simulink model "mathmodelsim"  (R2024b)
settings: Solver=VariableStepAuto  StartTime=0.0  StopTime=10  RelTol=1e-3
undefined symbols (not defined in the file): angles, initial_height, jointstiffnes_damping, limits, plane_x, plane_y, plane_z, torque, X, Y, Z
libraries: sm_lib x162, nesl_utility x70, simulink x9, rllib x1
(part 1 of 5)
settings Model: Creator=User  LastModifiedBy=User

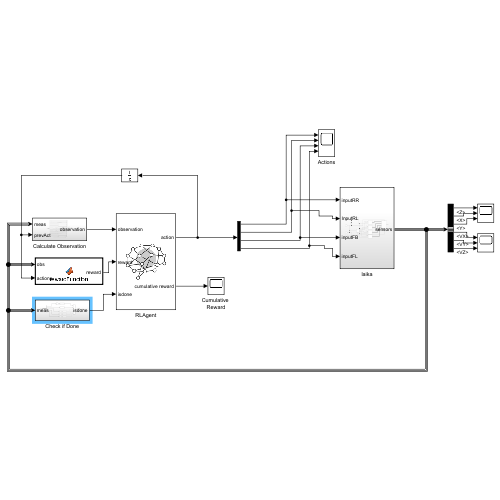
[thumbnail: Simulink's stored preview of the top-level diagram]
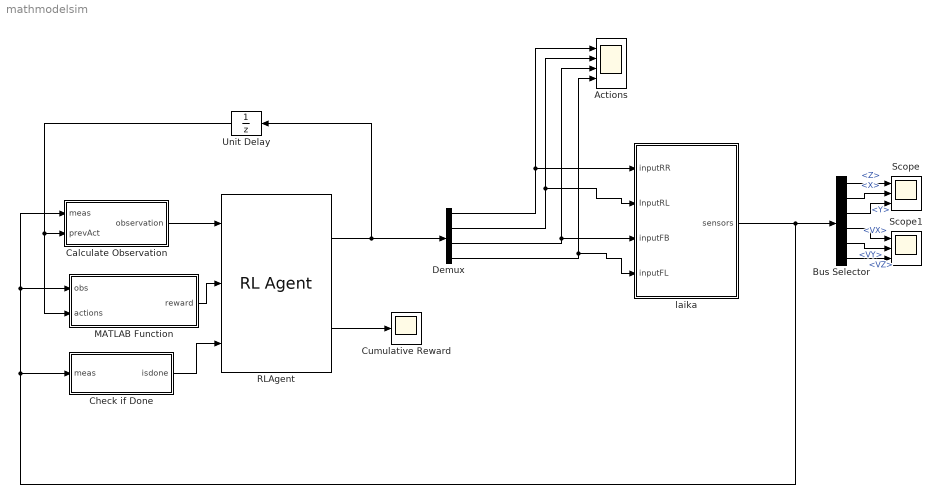
== system mathmodelsim ==
  Actions : Scope  NumInputPorts=4
  Bus Selector : BusSelector  OutputSignals=Z,X,Y,VX,VY,VZ
  Calculate Observation : Subsystem
  Check if Done : Subsystem
  Cumulative Reward : Scope
  Demux : Demux
  MATLAB Function : MATLAB Function  TreatAsAtomicUnit=on
  RLAgent : rllib/RL Agent  Agent=agent  ExternalActionAsInput=off  ProvideLastAction=off  ProvideCumRwd=on  TreatAsDirectFeedthrough=on  UseStrictObservationDataTypes=off
  Scope : Scope  NumInputPorts=3
  Scope1 : Scope  NumInputPorts=3
  Unit Delay : UnitDelay  SampleTime=-1  HasFrameUpgradeWarning=on
  laika : Subsystem
  wires:
  Bus Selector/1 -> Scope/1  "<Z>"
  Bus Selector/2 -> Scope/2  "<X>"
  Bus Selector/3 -> Scope/3  "<Y>"
  Bus Selector/4 -> Scope1/1  "<VX>"
  Bus Selector/5 -> Scope1/2  "<VY>"
  Bus Selector/6 -> Scope1/3  "<VZ>"
  Demux/3 -> Actions/3, laika/3(inputFB)
  RLAgent/2 -> Cumulative Reward/1
  Demux/2 -> laika/2(InputRL), Actions/2
  Demux/1 -> laika/1(inputRR), Actions/1
  Unit Delay/1 -> MATLAB Function/2(actions), Calculate Observation/2(prevAct)
  Demux/4 -> laika/4(inputFL), Actions/4
  MATLAB Function/1(reward) -> RLAgent/2
  Check if Done/1(isdone) -> RLAgent/3
  Calculate Observation/1(observation) -> RLAgent/1
  laika/1(sensors) -> Calculate Observation/1(meas), MATLAB Function/1(obs), Check if Done/1(meas), Bus Selector/1
  RLAgent/1 -> Demux/1, Unit Delay/1

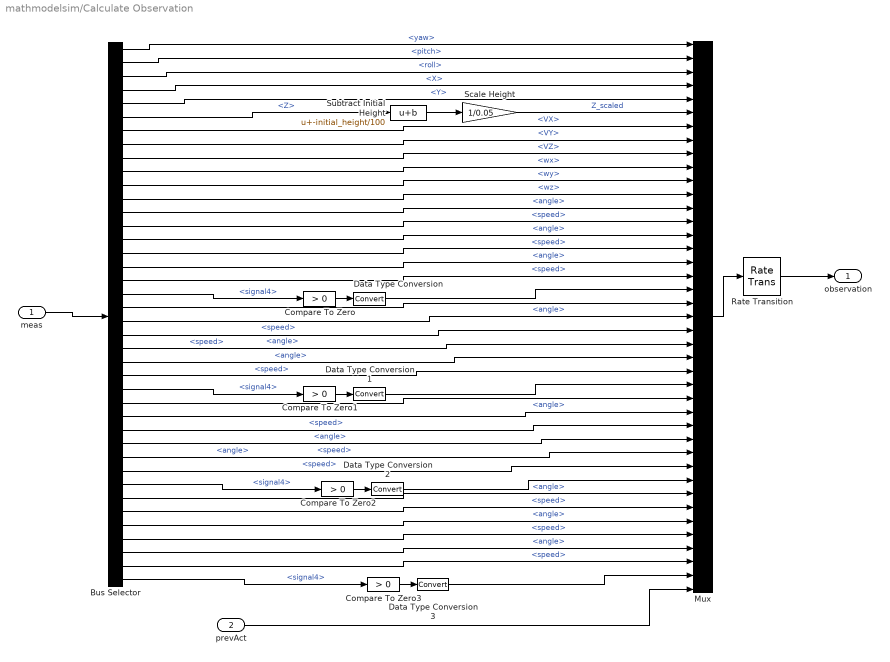
== system mathmodelsim/Calculate Observation ==
  meas : Inport
  prevAct : Inport  Port=2
  Bus Selector : BusSelector  OutputSignals=yaw,pitch,roll,X,Y,Z,VX,VY,VZ,wx,wy,wz,measRF.signal1.angle,measRF.signal1.speed,measRF.signal2.angle,measRF.signal2.speed,measRF.signal3.angle,measRF.signal3.speed,measRF.signal4,measRB.signal1.angle,measRB.signal1.speed,measRB.signal2.angle,measRB.signal2.speed,measRB.signal3.angle,measRB.signal3.speed,measRB.signal4,measLF.signal1.angle,measLF.signal1.speed,measLF.signal2.angle,measLF.signal2.speed,measLF.signal3.angle,measLF.signal3.speed,measLF.signal4,measLB.signal1.angle,measLB.signal1.speed,measLB.signal2.angle,measLB.signal2.speed,measLB.signal3.angle,measLB.signal3.speed,measLB.signal4
  Compare To Zero{,1..3} (4 alike) : simulink/Logic and Bit Operations/Compare To Zero  relop=>  OutDataTypeStr=boolean
  Data Type Conversion{,1..3} (4 alike) : DataTypeConversion  SaturateOnIntegerOverflow=off  RndMeth=Floor
  Mux : Mux  Inputs=41
  Rate Transition : RateTransition
  Scale Height : Gain  Gain=1/0.05
  Subtract Initial Height : Bias  Bias=-initial_height/100
  observation : Outport  VectorParamsAs1DForOutWhenUnconnected=off
  wires:
  Mux/1 -> Rate Transition/1
  Rate Transition/1 -> observation/1
  Bus Selector/1 -> Mux/1  "<yaw>"
  Bus Selector/2 -> Mux/2  "<pitch>"
  Bus Selector/3 -> Mux/3  "<roll>"
  Bus Selector/4 -> Mux/4  "<X>"
  Bus Selector/5 -> Mux/5  "<Y>"
  Bus Selector/7 -> Mux/7  "<VX>"
  Bus Selector/8 -> Mux/8  "<VY>"
  Bus Selector/9 -> Mux/9  "<VZ>"
  Bus Selector/10 -> Mux/10  "<wx>"
  Bus Selector/11 -> Mux/11  "<wy>"
  Bus Selector/12 -> Mux/12  "<wz>"
  Bus Selector/13 -> Mux/13  "<angle>"
  Bus Selector/14 -> Mux/14  "<speed>"
  Bus Selector/15 -> Mux/15  "<angle>"
  Bus Selector/16 -> Mux/16  "<speed>"
  Bus Selector/24 -> Mux/24  "<angle>"
  Bus Selector/17 -> Mux/17  "<angle>"
  Bus Selector/18 -> Mux/18  "<speed>"
  Bus Selector/20 -> Mux/20  "<angle>"
  Bus Selector/21 -> Mux/21  "<speed>"
  Bus Selector/22 -> Mux/22  "<angle>"
  Bus Selector/23 -> Mux/23  "<speed>"
  Bus Selector/25 -> Mux/25  "<speed>"
  Bus Selector/27 -> Mux/27  "<angle>"
  Bus Selector/28 -> Mux/28  "<speed>"
  Bus Selector/29 -> Mux/29  "<angle>"
  Bus Selector/30 -> Mux/30  "<speed>"
  Bus Selector/31 -> Mux/31  "<angle>"
  Bus Selector/32 -> Mux/32  "<speed>"
  Bus Selector/34 -> Mux/34  "<angle>"
  Bus Selector/35 -> Mux/35  "<speed>"
  Bus Selector/36 -> Mux/36  "<angle>"
  Bus Selector/37 -> Mux/37  "<speed>"
  Bus Selector/38 -> Mux/38  "<angle>"
  Bus Selector/39 -> Mux/39  "<speed>"
  prevAct/1 -> Mux/41
  Subtract Initial Height/1 -> Scale Height/1
  Bus Selector/6 -> Subtract Initial Height/1  "<Z>"
  Scale Height/1 -> Mux/6  "Z_scaled"
  Compare To Zero/1 -> Data Type Conversion/1
  Bus Selector/19 -> Compare To Zero/1  "<signal4>"
  Data Type Conversion/1 -> Mux/19
  Compare To Zero1/1 -> Data Type Conversion1/1
  Bus Selector/26 -> Compare To Zero1/1  "<signal4>"
  Data Type Conversion1/1 -> Mux/26
  Compare To Zero2/1 -> Data Type Conversion2/1
  Bus Selector/33 -> Compare To Zero2/1  "<signal4>"
  Data Type Conversion2/1 -> Mux/33
  Compare To Zero3/1 -> Data Type Conversion3/1
  Bus Selector/40 -> Compare To Zero3/1  "<signal4>"
  Data Type Conversion3/1 -> Mux/40
  meas/1 -> Bus Selector/1

== system mathmodelsim/Check if Done ==
  meas : Inport
  Abs : Abs  Commented=on  SaturateOnIntegerOverflow=off
  Abs1 : Abs  Commented=on  SaturateOnIntegerOverflow=off
  Abs2 : Abs  Commented=on  SaturateOnIntegerOverflow=off
  Abs3 : Abs  SaturateOnIntegerOverflow=off
  Bus Selector : BusSelector  OutputSignals=Y,Z,roll,pitch,yaw
  Compare To Constant : simulink/Logic and Bit Operations/Compare To Constant  Commented=on  relop=>=  const=pi/4  OutDataTypeStr=boolean
  Compare To Constant1 : simulink/Logic and Bit Operations/Compare To Constant  Commented=on  relop=>=  const=pi/4  OutDataTypeStr=boolean
  Compare To Constant2 : simulink/Logic and Bit Operations/Compare To Constant  Commented=on  relop=>=  const=pi/4  OutDataTypeStr=boolean
  Detect Fallen Robot : simulink/Logic and Bit Operations/Compare To Constant  relop=<=  const=0.3  OutDataTypeStr=boolean
  Detect Lateral Motion : simulink/Logic and Bit Operations/Compare To Constant  relop=>  const=0.7  OutDataTypeStr=boolean
  Logical Operator : Logic  Operator=OR  Inputs=5  AllPortsSameDT=off  OutDataTypeStr=boolean
  Rate Transition : RateTransition
  isdone : Outport  VectorParamsAs1DForOutWhenUnconnected=off
  wires:
  Logical Operator/1 -> Rate Transition/1
  Bus Selector/2 -> Detect Fallen Robot/1  "<Z>"
  Detect Fallen Robot/1 -> Logical Operator/2
  Bus Selector/3 -> Abs/1  "<roll>"
  Bus Selector/4 -> Abs1/1  "<pitch>"
  Compare To Constant/1 -> Logical Operator/3
  Abs/1 -> Compare To Constant/1
  Abs1/1 -> Compare To Constant1/1
  Compare To Constant1/1 -> Logical Operator/4
  Rate Transition/1 -> isdone/1
  Abs2/1 -> Compare To Constant2/1
  Bus Selector/5 -> Abs2/1  "<yaw>"
  Compare To Constant2/1 -> Logical Operator/5
  Abs3/1 -> Detect Lateral Motion/1
  Bus Selector/1 -> Abs3/1  "<Y>"
  Detect Lateral Motion/1 -> Logical Operator/1
  meas/1 -> Bus Selector/1

== system mathmodelsim/laika ==
  inputRR : Inport
  InputRL : Inport  Port=2
  inputFB : Inport  Port=3
  inputFL : Inport  Port=4
  MechanismConfiguration : sm_lib/Utilities/Mechanism Configuration  UniformGravity=Constant  GravityVector=[0 0 -9.80665]  GravityVectorUnits=m/s^2  LinearizationDelta=0.001  JointModeTransitionNonlinearIterations=2
  RL : Subsystem
  RR : Subsystem
  Sensors : Subsystem
      settings: PortSchema="{\"entries\":[{\"content\":{\"sides\":[{\"content\":{\"connectorIds\":[\"In1\",\"In2\",\"In3\",\"In4\"]},\"type\":\"ConnectorPlacement.EquallySpacedRectSide\",\"uuid\":\"3df3d218-abd4-4704-a7f5-393c9b3793f0\"},{\"content\":{\"connectorIds\":[\"Out1\"],\"side\":\"RIGHT\"},\"type\":\"ConnectorPlacement.EquallySpacedRectSide\",\"uuid\":\"04e38e81-ef79-4693-9892-346f49c2e321\"},{\"content\":{\"connectorIds\":[\"LConn1\"],\"side\":\"TOP\"},\"type\":\"ConnectorPlacement.EquallySpacedRectSide\",\"uuid\":\"c131dd2b-291e-43b4-b02f-8f9d4b7fd98b\"},{\"content\":{\"connectorIds\":[\"RConn1\"],\"side\":\"BOTTOM\"},\"type\":\"ConnectorPlacement.EquallySpacedRectSide\",\"uuid\":\"5d7f36dd-2d30-4e6e-ba6f-2e7b92d39c5b\"}]},\"type\":\"ConnectorPlacement.EquallySpacedConnector\",\"uuid\":\"032ee98f-9dac-462a-bb2a-479e479c13aa\"}],\"packageUris\":[\"http://schema.mathworks.com/mf0/Connector/R2020b\"],\"version\":\"1.0\"}"
  Solver Configuration : nesl_utility/Solver Configuration  PhysicalDomain=network_engine_domain  SubClassName=solver  LeftPortType=input  RightPortType=generic  Tones=[]  Harmonics=[]  SimulateNoise=off  Profile=off  UseLocalSampling=off  EnableSwitchedLinearOptims=on  FrequencyDomain=off  UseCCode=off  RelTol=0.001  AbsTol=0.001  MinStep=1e-09  ToWorkspace=off  RevertToSquareIcSolve=off  NumHomotopyIterations=100  PhasorMode=off  PhasorModeNumHarmonics=1  ConsistencySolver=NEWTON_XTOL_AFTER_FTOL  IndexReductionMethod=DerivativeReplacement  DoDC=off  ResidualTolerance=1e-09  ConsistencyTolSource=GLOBAL  ConsistencyAbsTol=0.001  ConsistencyRelTol=0.001  ConsistencyTolFactor=0.001  UseLocalSolver=off  LocalSolverChoice=NE_BACKWARD_EULER_ADVANCER  ResolveIndetEquations=on  FunctionEvalNumThread=1  LocalSolverSampleTime=0.001  DoFixedCost=off  MaxNonlinIter=3  MaxModeIter=2  ComputeImpulses=off  ImpulseIterations=2  LinearAlgebra=auto  LinearAlgebraNumThread=0  EquationFormulation=NE_TIME_EF  DelaysMemoryBudget=1024  AutomaticFiltering=on  FilteringTimeConstant=0.001  PartitionStorageMethod=AS_NEEDED  PartitionMemoryBudget=1024  PartitionMethod=ROBUST  MultibodyUseLocalSolver=off  MultibodyLocalSolverChoice=ODE1  MultibodyLocalSolverSampleTime=0.001
  Subsystem : Subsystem
  Subsystem1 : Subsystem
  World : sm_lib/Frames and Transforms/World Frame
  World Plane : sm_lib/Body Elements/Brick Solid  BrickDimensions=[plane_x plane_y plane_z]  BrickDimensionsUnits=m  ExportEntireGeometry=on  InertiaType=CalculateFromGeometry  BasedOnType=Density  Density=1000  DensityUnits=kg/(m^3)  Mass=1  MassUnits=kg  CenterOfMass=[0 0 0]  CenterOfMassUnits=m  MomentsOfInertia=[1 1 1]  MomentsOfInertiaUnits=kg*m^2  ProductsOfInertia=[0 0 0]  ProductsOfInertiaUnits=kg*m^2  GraphicType=FromGeometry  MarkerShape=Sphere  MarkerSize=10  GraphicVisPropType=SimpleVisualProperties  GraphicDiffuseColor=[0.05882 1 1]  GraphicOpacity=0.5  GraphicSpecularColor=[0.5 0.5 0.5 1.0]  GraphicAmbientColor=[0.15 0.15 0.15 1.0]  GraphicEmissiveColor=[0.0 0.0 0.0 1.0]  GraphicShininess=75  DoExposeReferenceFrame=on  SerializedFrames=<Frames/>
  chassis : Subsystem
      settings: PortSchema="{\"entries\":[{\"content\":{\"sides\":[{\"content\":{\"connectorIds\":[\"LConn1\"]},\"type\":\"ConnectorPlacement.EquallySpacedRectSide\",\"uuid\":\"e8b07a4b-cdda-468b-a417-21e1e893ca66\"},{\"content\":{\"connectorIds\":[\"RConn1\",\"RConn2\",\"RConn3\",\"RConn4\"],\"side\":\"RIGHT\"},\"type\":\"ConnectorPlacement.EquallySpacedRectSide\",\"uuid\":\"0565d4ec-0cbc-4c5e-bd83-3e7a8f475fde\"},{\"content\":{\"side\":\"TOP\"},\"type\":\"ConnectorPlacement.EquallySpacedRectSide\",\"uuid\":\"c3232b26-b645-4cd2-920f-d5223db3508f\"},{\"content\":{\"connectorIds\":[\"RConn5\"],\"side\":\"BOTTOM\"},\"type\":\"ConnectorPlacement.EquallySpacedRectSide\",\"uuid\":\"50ebb0e1-0afe-400d-9193-05a5ee19282a\"}]},\"type\":\"ConnectorPlacement.EquallySpacedConnector\",\"uuid\":\"88d54b84-644a-4a43-8038-ee8ee609d3c5\"}],\"packageUris\":[\"http://schema.mathworks.com/mf0/Connector/R2020b\"],\"version\":\"1.0\"}"
  offset : sm_lib/Frames and Transforms/Rigid Transform  RotationMethod=RotationSequence  FollAlignAxisA=+X  BaseAlignAxisA=+Y  FollAlignAxisB=+Y  BaseAlignAxisB=+Z  RotationStandardAxis=+Z  RotationAngle=0  RotationAngleUnits=deg  RotationArbitraryAxis=[0 0 1]  RotationSequenceAxes=BaseAxes  RotationSequence=XYZ  RotationSequenceAngles=[0, 0, 0]  RotationSequenceAnglesUnits=rad  RotationMatrix=[1 0 0;0 1 0;0 0 1]  Quaternion=[1 0 0 0]  TranslationMethod=Cartesian  TranslationCartesianOffset=[0, 0, -0.1]  TranslationCartesianOffsetUnits=m  TranslationStandardAxis=+Z  TranslationStandardOffset=0  TranslationStandardOffsetUnits=m  TranslationROffset=0  TranslationROffsetUnits=m  TranslationThetaOffset=0  TranslationThetaOffsetUnits=deg  TranslationZOffset=0  TranslationZOffsetUnits=m
  sensors : Outport
  wires:
  Subsystem/1(meas) -> Sensors/3(measFB)
  Sensors/1(sensors) -> sensors/1
  Subsystem1/1(meas) -> Sensors/4(measFL)
  InputRL/1 -> RL/1(InputRL)
  inputFL/1 -> Subsystem1/1(InputFL)
  RR/1(meas) -> Sensors/1(measRR)
  inputFB/1 -> Subsystem/1(InputFB)
  RL/1(meas) -> Sensors/2(measRL)
  inputRR/1 -> RR/1(InputRR)
  connections:
  MechanismConfiguration/RConn1 -- Solver Configuration/RConn1 -- Sensors/LConn1 -- offset/RConn1 -- World/RConn1 -- chassis/LConn1
  World Plane/LConn1 -- RR/LConn2 -- RL/LConn2 -- Subsystem1/LConn2 -- Subsystem/LConn2
  chassis/RConn4 -- Subsystem1/LConn1
  RR/LConn1 -- chassis/RConn1
  Subsystem/LConn1 -- chassis/RConn3
  chassis/RConn5 -- Sensors/RConn1
  chassis/RConn2 -- RL/LConn1
  World Plane/RConn1 -- offset/LConn1

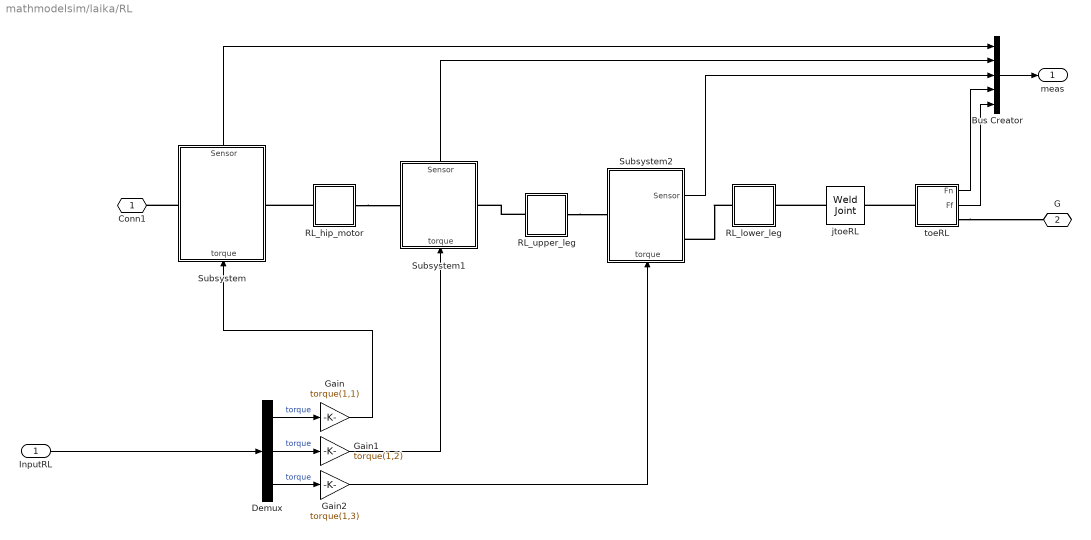
== system mathmodelsim/laika/RL ==
  InputRL : Inport
  Bus Creator : BusCreator  Inputs=5
  Demux : Demux  Outputs=3
  Gain : Gain  Gain=torque(1,1)
  Gain1 : Gain  Gain=torque(1,2)
  Gain2 : Gain  Gain=torque(1,3)
  RL_hip_motor : Subsystem
  RL_lower_leg : Subsystem
  RL_upper_leg : Subsystem
  Subsystem : Subsystem
      settings: PortSchema="{\"entries\":[{\"content\":{\"sides\":[{\"content\":{\"connectorIds\":[\"LConn1\"]},\"type\":\"ConnectorPlacement.EquallySpacedRectSide\",\"uuid\":\"d10d1646-662a-418c-8f44-f8cb7d7b2586\"},{\"content\":{\"connectorIds\":[\"RConn1\"],\"side\":\"RIGHT\"},\"type\":\"ConnectorPlacement.EquallySpacedRectSide\",\"uuid\":\"1df4eb92-be91-4006-ac5e-dec2e273d2b2\"},{\"content\":{\"connectorIds\":[\"Out1\"],\"side\":\"TOP\"},\"type\":\"ConnectorPlacement.EquallySpacedRectSide\",\"uuid\":\"1cbb86fd-02d7-4865-80eb-cfab46dca279\"},{\"content\":{\"connectorIds\":[\"In1\"],\"side\":\"BOTTOM\"},\"type\":\"ConnectorPlacement.EquallySpacedRectSide\",\"uuid\":\"c11095bb-d672-4e30-a4ef-8f5c7235aabe\"}]},\"type\":\"ConnectorPlacement.EquallySpacedConnector\",\"uuid\":\"62703e30-84e5-4f8f-9fd6-529661229832\"}],\"packageUris\":[\"http://schema.mathworks.com/mf0/Connector/R2020b\"],\"version\":\"1.0\"}"
  Subsystem1 : Subsystem
      settings: PortSchema="{\"entries\":[{\"content\":{\"sides\":[{\"content\":{\"connectorIds\":[\"LConn1\"]},\"type\":\"ConnectorPlacement.EquallySpacedRectSide\",\"uuid\":\"d10d1646-662a-418c-8f44-f8cb7d7b2586\"},{\"content\":{\"connectorIds\":[\"RConn1\"],\"side\":\"RIGHT\"},\"type\":\"ConnectorPlacement.EquallySpacedRectSide\",\"uuid\":\"1df4eb92-be91-4006-ac5e-dec2e273d2b2\"},{\"content\":{\"connectorIds\":[\"Out1\"],\"side\":\"TOP\"},\"type\":\"ConnectorPlacement.EquallySpacedRectSide\",\"uuid\":\"1cbb86fd-02d7-4865-80eb-cfab46dca279\"},{\"content\":{\"connectorIds\":[\"In1\"],\"side\":\"BOTTOM\"},\"type\":\"ConnectorPlacement.EquallySpacedRectSide\",\"uuid\":\"8bee2df4-a927-4cf9-9983-bdcad833a156\"}]},\"type\":\"ConnectorPlacement.EquallySpacedConnector\",\"uuid\":\"62703e30-84e5-4f8f-9fd6-529661229832\"}],\"packageUris\":[\"http://schema.mathworks.com/mf0/Connector/R2020b\"],\"version\":\"1.0\"}"
  Subsystem2 : Subsystem
      settings: PortSchema="{\"entries\":[{\"content\":{\"sides\":[{\"content\":{\"connectorIds\":[\"LConn1\"]},\"type\":\"ConnectorPlacement.EquallySpacedRectSide\",\"uuid\":\"d10d1646-662a-418c-8f44-f8cb7d7b2586\"},{\"content\":{\"connectorIds\":[\"Out1\",\"RConn1\"],\"side\":\"RIGHT\"},\"type\":\"ConnectorPlacement.EquallySpacedRectSide\",\"uuid\":\"1df4eb92-be91-4006-ac5e-dec2e273d2b2\"},{\"content\":{\"side\":\"TOP\"},\"type\":\"ConnectorPlacement.EquallySpacedRectSide\",\"uuid\":\"1cbb86fd-02d7-4865-80eb-cfab46dca279\"},{\"content\":{\"connectorIds\":[\"In1\"],\"side\":\"BOTTOM\"},\"type\":\"ConnectorPlacement.EquallySpacedRectSide\",\"uuid\":\"666c5156-ac3a-4b1c-905d-ea8e134facab\"}]},\"type\":\"ConnectorPlacement.EquallySpacedConnector\",\"uuid\":\"62703e30-84e5-4f8f-9fd6-529661229832\"}],\"packageUris\":[\"http://schema.mathworks.com/mf0/Connector/R2020b\"],\"version\":\"1.0\"}"
  jtoeRL : sm_lib/Joints/Weld Joint  JointMode=Normal  CompositeWrenchDir=FollowerOnBase  CompositeWrenchFrame=BaseFrame  SenseConstraintForce=off  SenseConstraintTorque=off  SenseTotalForce=off  SenseTotalTorque=off
  toeRL : Subsystem
  Conn1 : PMIOPort  Side=Left
  G : PMIOPort  Port=2  Side=Left
  meas : Outport  VectorParamsAs1DForOutWhenUnconnected=off
  wires:
  Bus Creator/1 -> meas/1
  toeRL/1(Fn) -> Bus Creator/4
  toeRL/2(Ff) -> Bus Creator/5
  Subsystem/1(Sensor) -> Bus Creator/1
  Subsystem1/1(Sensor) -> Bus Creator/2
  Subsystem2/1(Sensor) -> Bus Creator/3
  Gain2/1 -> Subsystem2/1(torque)
  InputRL/1 -> Demux/1
  Demux/1 -> Gain/1  "torque"
  Demux/2 -> Gain1/1  "torque"
  Demux/3 -> Gain2/1  "torque"
  Gain1/1 -> Subsystem1/1(torque)
  Gain/1 -> Subsystem/1(torque)
  connections:
  toeRL/LConn1 -- jtoeRL/RConn1
  jtoeRL/LConn1 -- RL_lower_leg/RConn1
  Subsystem/LConn1 -- Conn1/RConn1
  RL_hip_motor/LConn1 -- Subsystem/RConn1
  toeRL/RConn1 -- G/RConn1
  RL_upper_leg/LConn1 -- Subsystem1/RConn1
  RL_hip_motor/RConn1 -- Subsystem1/LConn1
  RL_upper_leg/RConn1 -- Subsystem2/LConn1
  RL_lower_leg/LConn1 -- Subsystem2/RConn1

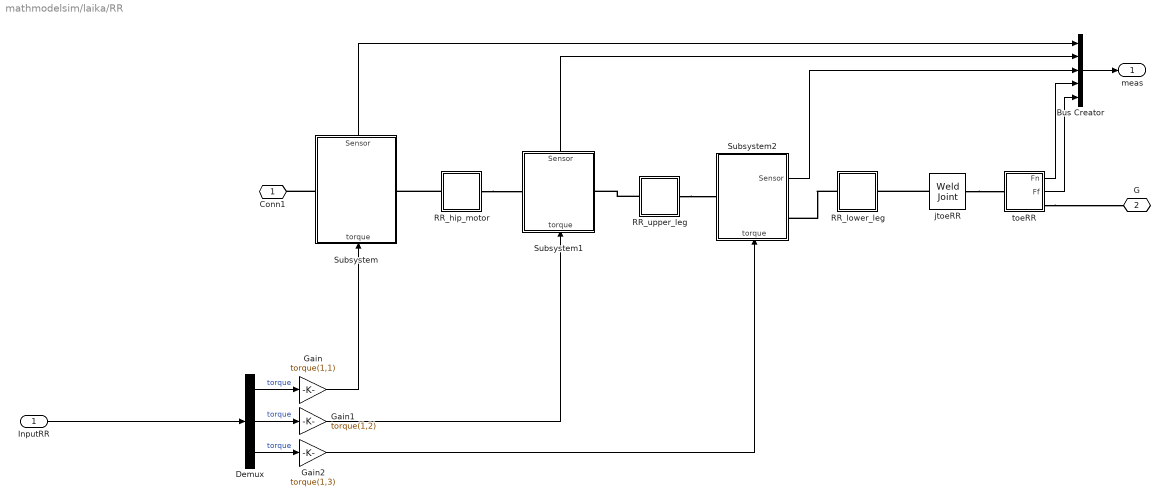
== system mathmodelsim/laika/RR ==
  InputRR : Inport
  Bus Creator : BusCreator  Inputs=5
  Demux : Demux  Outputs=3
  Gain : Gain  Gain=torque(1,1)
  Gain1 : Gain  Gain=torque(1,2)
  Gain2 : Gain  Gain=torque(1,3)
  RR_hip_motor : Subsystem
  RR_lower_leg : Subsystem
  RR_upper_leg : Subsystem
  Subsystem : Subsystem
      settings: PortSchema="{\"entries\":[{\"content\":{\"sides\":[{\"content\":{\"connectorIds\":[\"LConn1\"]},\"type\":\"ConnectorPlacement.EquallySpacedRectSide\",\"uuid\":\"d10d1646-662a-418c-8f44-f8cb7d7b2586\"},{\"content\":{\"connectorIds\":[\"RConn1\"],\"side\":\"RIGHT\"},\"type\":\"ConnectorPlacement.EquallySpacedRectSide\",\"uuid\":\"1df4eb92-be91-4006-ac5e-dec2e273d2b2\"},{\"content\":{\"connectorIds\":[\"Out1\"],\"side\":\"TOP\"},\"type\":\"ConnectorPlacement.EquallySpacedRectSide\",\"uuid\":\"1cbb86fd-02d7-4865-80eb-cfab46dca279\"},{\"content\":{\"connectorIds\":[\"In1\"],\"side\":\"BOTTOM\"},\"type\":\"ConnectorPlacement.EquallySpacedRectSide\",\"uuid\":\"c11095bb-d672-4e30-a4ef-8f5c7235aabe\"}]},\"type\":\"ConnectorPlacement.EquallySpacedConnector\",\"uuid\":\"62703e30-84e5-4f8f-9fd6-529661229832\"}],\"packageUris\":[\"http://schema.mathworks.com/mf0/Connector/R2020b\"],\"version\":\"1.0\"}"
  Subsystem1 : Subsystem
      settings: PortSchema="{\"entries\":[{\"content\":{\"sides\":[{\"content\":{\"connectorIds\":[\"LConn1\"]},\"type\":\"ConnectorPlacement.EquallySpacedRectSide\",\"uuid\":\"d10d1646-662a-418c-8f44-f8cb7d7b2586\"},{\"content\":{\"connectorIds\":[\"RConn1\"],\"side\":\"RIGHT\"},\"type\":\"ConnectorPlacement.EquallySpacedRectSide\",\"uuid\":\"1df4eb92-be91-4006-ac5e-dec2e273d2b2\"},{\"content\":{\"connectorIds\":[\"Out1\"],\"side\":\"TOP\"},\"type\":\"ConnectorPlacement.EquallySpacedRectSide\",\"uuid\":\"1cbb86fd-02d7-4865-80eb-cfab46dca279\"},{\"content\":{\"connectorIds\":[\"In1\"],\"side\":\"BOTTOM\"},\"type\":\"ConnectorPlacement.EquallySpacedRectSide\",\"uuid\":\"8bee2df4-a927-4cf9-9983-bdcad833a156\"}]},\"type\":\"ConnectorPlacement.EquallySpacedConnector\",\"uuid\":\"62703e30-84e5-4f8f-9fd6-529661229832\"}],\"packageUris\":[\"http://schema.mathworks.com/mf0/Connector/R2020b\"],\"version\":\"1.0\"}"
  Subsystem2 : Subsystem
      settings: PortSchema="{\"entries\":[{\"content\":{\"sides\":[{\"content\":{\"connectorIds\":[\"LConn1\"]},\"type\":\"ConnectorPlacement.EquallySpacedRectSide\",\"uuid\":\"d10d1646-662a-418c-8f44-f8cb7d7b2586\"},{\"content\":{\"connectorIds\":[\"Out1\",\"RConn1\"],\"side\":\"RIGHT\"},\"type\":\"ConnectorPlacement.EquallySpacedRectSide\",\"uuid\":\"1df4eb92-be91-4006-ac5e-dec2e273d2b2\"},{\"content\":{\"side\":\"TOP\"},\"type\":\"ConnectorPlacement.EquallySpacedRectSide\",\"uuid\":\"1cbb86fd-02d7-4865-80eb-cfab46dca279\"},{\"content\":{\"connectorIds\":[\"In1\"],\"side\":\"BOTTOM\"},\"type\":\"ConnectorPlacement.EquallySpacedRectSide\",\"uuid\":\"666c5156-ac3a-4b1c-905d-ea8e134facab\"}]},\"type\":\"ConnectorPlacement.EquallySpacedConnector\",\"uuid\":\"62703e30-84e5-4f8f-9fd6-529661229832\"}],\"packageUris\":[\"http://schema.mathworks.com/mf0/Connector/R2020b\"],\"version\":\"1.0\"}"
  jtoeRR : sm_lib/Joints/Weld Joint  JointMode=Normal  CompositeWrenchDir=FollowerOnBase  CompositeWrenchFrame=BaseFrame  SenseConstraintForce=off  SenseConstraintTorque=off  SenseTotalForce=off  SenseTotalTorque=off
  toeRR : Subsystem
  Conn1 : PMIOPort  Side=Left
  G : PMIOPort  Port=2  Side=Left
  meas : Outport  VectorParamsAs1DForOutWhenUnconnected=off
  wires:
  Bus Creator/1 -> meas/1
  toeRR/1(Fn) -> Bus Creator/4
  toeRR/2(Ff) -> Bus Creator/5
  Subsystem/1(Sensor) -> Bus Creator/1
  Demux/3 -> Gain2/1  "torque"
  InputRR/1 -> Demux/1
  Demux/2 -> Gain1/1  "torque"
  Demux/1 -> Gain/1  "torque"
  Subsystem1/1(Sensor) -> Bus Creator/2
  Subsystem2/1(Sensor) -> Bus Creator/3
  Gain/1 -> Subsystem/1(torque)
  Gain1/1 -> Subsystem1/1(torque)
  Gain2/1 -> Subsystem2/1(torque)
  connections:
  jtoeRR/RConn1 -- toeRR/LConn1
  jtoeRR/LConn1 -- RR_lower_leg/RConn1
  Subsystem/LConn1 -- Conn1/RConn1
  RR_hip_motor/LConn1 -- Subsystem/RConn1
  toeRR/RConn1 -- G/RConn1
  RR_upper_leg/LConn1 -- Subsystem1/RConn1
  RR_hip_motor/RConn1 -- Subsystem1/LConn1
  RR_upper_leg/RConn1 -- Subsystem2/LConn1
  RR_lower_leg/LConn1 -- Subsystem2/RConn1

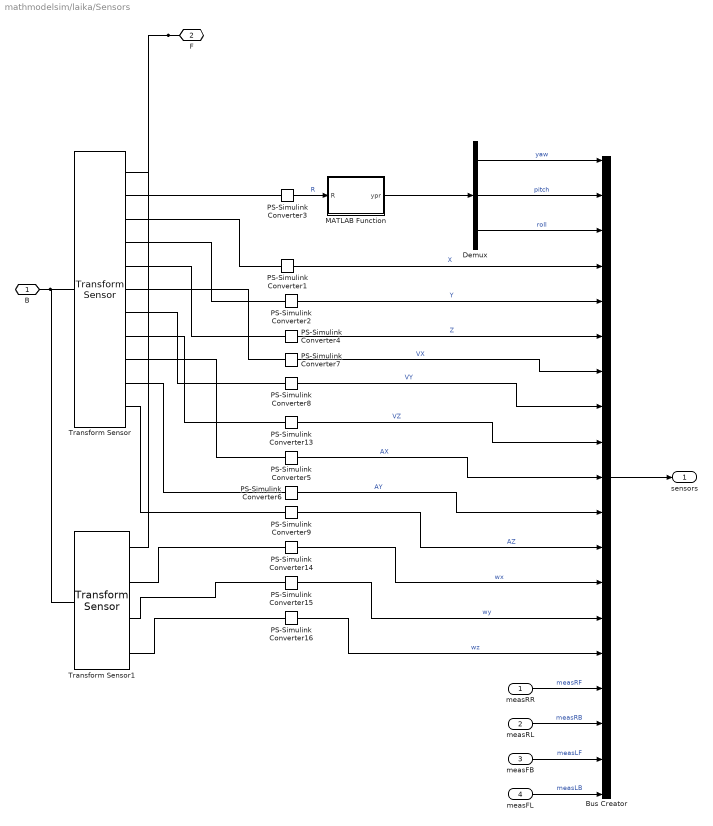
== system mathmodelsim/laika/Sensors ==
  measRR : Inport
  measRL : Inport  Port=2
  measFB : Inport  Port=3
  measFL : Inport  Port=4
  Bus Creator : BusCreator  Inputs=19
  Demux : Demux  Outputs=3
  MATLAB Function : MATLAB Function  TreatAsAtomicUnit=on
  PS-Simulink Converter{1..9,13..16} (13 alike) : nesl_utility/PS-Simulink Converter  PhysicalDomain=network_engine_domain  SubClassName=ps_output  LeftPortType=input  RightPortType=output  PseudoPeriodic=off  Frequencies=[]  VectorFormat=1-D array  Unit=1  AffineConversion=off
  Transform Sensor : sm_lib/Frames and Transforms/Transform Sensor  MeasurementFrame=World  RotationSequence=XYX  SenseAngle=off  SenseAxis=off  SenseQ=off  SenseR=on  SenseRotationSequence=off  SenseOmegaX=off  SenseOmegaY=off  SenseOmegaZ=off  SenseOmega=off  SenseQDot=off  SenseRDot=off  SenseRotationSequenceDot=off  SenseAlphaX=off  SenseAlphaY=off  SenseAlphaZ=off  SenseAlpha=off  SenseQDDot=off  SenseRDDot=off  SenseX=on  SenseY=on  SenseZ=on  SenseXYZ=off  SenseRad=off  SenseAzim=off  SenseDist=off  SenseInc=off  SenseXDot=on  SenseYDot=on  SenseZDot=on  SenseXYZDot=off  SenseRadDot=off  SenseAzimDot=off  SenseDistDot=off  SenseIncDot=off  SenseXDDot=on  SenseYDDot=on  SenseZDDot=on  SenseXYZDDot=off  SenseRadDDot=off  SenseAzimDDot=off  SenseDistDDot=off  SenseIncDDot=off
  Transform Sensor1 : sm_lib/Frames and Transforms/Transform Sensor  MeasurementFrame=NonRotatingFollower  RotationSequence=XYX  SenseAngle=off  SenseAxis=off  SenseQ=off  SenseR=off  SenseRotationSequence=off  SenseOmegaX=on  SenseOmegaY=on  SenseOmegaZ=on  SenseOmega=off  SenseQDot=off  SenseRDot=off  SenseRotationSequenceDot=off  SenseAlphaX=off  SenseAlphaY=off  SenseAlphaZ=off  SenseAlpha=off  SenseQDDot=off  SenseRDDot=off  SenseX=off  SenseY=off  SenseZ=off  SenseXYZ=off  SenseRad=off  SenseAzim=off  SenseDist=off  SenseInc=off  SenseXDot=off  SenseYDot=off  SenseZDot=off  SenseXYZDot=off  SenseRadDot=off  SenseAzimDot=off  SenseDistDot=off  SenseIncDot=off  SenseXDDot=off  SenseYDDot=off  SenseZDDot=off  SenseXYZDDot=off  SenseRadDDot=off  SenseAzimDDot=off  SenseDistDDot=off  SenseIncDDot=off
  B : PMIOPort  Side=Left
  F : PMIOPort  Port=2  Side=Right
  sensors : Outport  VectorParamsAs1DForOutWhenUnconnected=off
  wires:
  measRL/1 -> Bus Creator/17  "measRB"
  PS-Simulink Converter14/1 -> Bus Creator/13  "wx"
  PS-Simulink Converter15/1 -> Bus Creator/14  "wy"
  Demux/3 -> Bus Creator/3  "roll"
  Bus Creator/1 -> sensors/1
  PS-Simulink Converter9/1 -> Bus Creator/12  "AZ"
  PS-Simulink Converter7/1 -> Bus Creator/7  "VX"
  PS-Simulink Converter8/1 -> Bus Creator/8  "VY"
  Demux/2 -> Bus Creator/2  "pitch"
  PS-Simulink Converter13/1 -> Bus Creator/9  "VZ"
  PS-Simulink Converter4/1 -> Bus Creator/6  "Z"
  Demux/1 -> Bus Creator/1  "yaw"
  measRR/1 -> Bus Creator/16  "measRF"
  PS-Simulink Converter5/1 -> Bus Creator/10  "AX"
  PS-Simulink Converter6/1 -> Bus Creator/11  "AY"
  MATLAB Function/1(ypr) -> Demux/1
  PS-Simulink Converter1/1 -> Bus Creator/4  "X"
  PS-Simulink Converter16/1 -> Bus Creator/15  "wz"
  PS-Simulink Converter2/1 -> Bus Creator/5  "Y"
  PS-Simulink Converter3/1 -> MATLAB Function/1(R)  "R"
  measFB/1 -> Bus Creator/18  "measLF"
  measFL/1 -> Bus Creator/19  "measLB"
  connections:
  F/RConn1 -- Transform Sensor/RConn1 -- Transform Sensor1/RConn1
  B/RConn1 -- Transform Sensor/LConn1 -- Transform Sensor1/LConn1
  PS-Simulink Converter13/LConn1 -- Transform Sensor/RConn8
  Transform Sensor/RConn10 -- PS-Simulink Converter6/LConn1
  Transform Sensor/RConn4 -- PS-Simulink Converter2/LConn1
  Transform Sensor/RConn5 -- PS-Simulink Converter4/LConn1
  Transform Sensor1/RConn4 -- PS-Simulink Converter16/LConn1
  Transform Sensor/RConn7 -- PS-Simulink Converter8/LConn1
  PS-Simulink Converter14/LConn1 -- Transform Sensor1/RConn2
  PS-Simulink Converter1/LConn1 -- Transform Sensor/RConn3
  PS-Simulink Converter15/LConn1 -- Transform Sensor1/RConn3
  PS-Simulink Converter5/LConn1 -- Transform Sensor/RConn9
  PS-Simulink Converter3/LConn1 -- Transform Sensor/RConn2
  PS-Simulink Converter7/LConn1 -- Transform Sensor/RConn6
  Transform Sensor/RConn11 -- PS-Simulink Converter9/LConn1

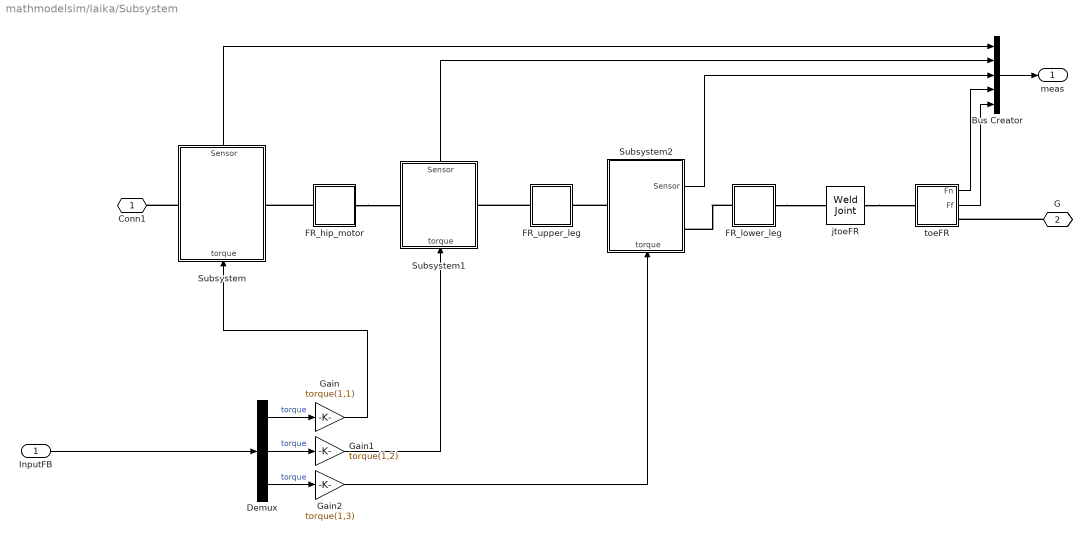
== system mathmodelsim/laika/Subsystem ==
  InputFB : Inport
  Bus Creator : BusCreator  Inputs=5
  Demux : Demux  Outputs=3
  FR_hip_motor : Subsystem
  FR_lower_leg : Subsystem
  FR_upper_leg : Subsystem
  Gain : Gain  Gain=torque(1,1)
  Gain1 : Gain  Gain=torque(1,2)
  Gain2 : Gain  Gain=torque(1,3)
  Subsystem : Subsystem
      settings: PortSchema="{\"entries\":[{\"content\":{\"sides\":[{\"content\":{\"connectorIds\":[\"LConn1\"]},\"type\":\"ConnectorPlacement.EquallySpacedRectSide\",\"uuid\":\"d10d1646-662a-418c-8f44-f8cb7d7b2586\"},{\"content\":{\"connectorIds\":[\"RConn1\"],\"side\":\"RIGHT\"},\"type\":\"ConnectorPlacement.EquallySpacedRectSide\",\"uuid\":\"1df4eb92-be91-4006-ac5e-dec2e273d2b2\"},{\"content\":{\"connectorIds\":[\"Out1\"],\"side\":\"TOP\"},\"type\":\"ConnectorPlacement.EquallySpacedRectSide\",\"uuid\":\"1cbb86fd-02d7-4865-80eb-cfab46dca279\"},{\"content\":{\"connectorIds\":[\"In1\"],\"side\":\"BOTTOM\"},\"type\":\"ConnectorPlacement.EquallySpacedRectSide\",\"uuid\":\"c11095bb-d672-4e30-a4ef-8f5c7235aabe\"}]},\"type\":\"ConnectorPlacement.EquallySpacedConnector\",\"uuid\":\"62703e30-84e5-4f8f-9fd6-529661229832\"}],\"packageUris\":[\"http://schema.mathworks.com/mf0/Connector/R2020b\"],\"version\":\"1.0\"}"
  Subsystem1 : Subsystem
      settings: PortSchema="{\"entries\":[{\"content\":{\"sides\":[{\"content\":{\"connectorIds\":[\"LConn1\"]},\"type\":\"ConnectorPlacement.EquallySpacedRectSide\",\"uuid\":\"d10d1646-662a-418c-8f44-f8cb7d7b2586\"},{\"content\":{\"connectorIds\":[\"RConn1\"],\"side\":\"RIGHT\"},\"type\":\"ConnectorPlacement.EquallySpacedRectSide\",\"uuid\":\"1df4eb92-be91-4006-ac5e-dec2e273d2b2\"},{\"content\":{\"connectorIds\":[\"Out1\"],\"side\":\"TOP\"},\"type\":\"ConnectorPlacement.EquallySpacedRectSide\",\"uuid\":\"1cbb86fd-02d7-4865-80eb-cfab46dca279\"},{\"content\":{\"connectorIds\":[\"In1\"],\"side\":\"BOTTOM\"},\"type\":\"ConnectorPlacement.EquallySpacedRectSide\",\"uuid\":\"8bee2df4-a927-4cf9-9983-bdcad833a156\"}]},\"type\":\"ConnectorPlacement.EquallySpacedConnector\",\"uuid\":\"62703e30-84e5-4f8f-9fd6-529661229832\"}],\"packageUris\":[\"http://schema.mathworks.com/mf0/Connector/R2020b\"],\"version\":\"1.0\"}"
  Subsystem2 : Subsystem
      settings: PortSchema="{\"entries\":[{\"content\":{\"sides\":[{\"content\":{\"connectorIds\":[\"LConn1\"]},\"type\":\"ConnectorPlacement.EquallySpacedRectSide\",\"uuid\":\"d10d1646-662a-418c-8f44-f8cb7d7b2586\"},{\"content\":{\"connectorIds\":[\"Out1\",\"RConn1\"],\"side\":\"RIGHT\"},\"type\":\"ConnectorPlacement.EquallySpacedRectSide\",\"uuid\":\"1df4eb92-be91-4006-ac5e-dec2e273d2b2\"},{\"content\":{\"side\":\"TOP\"},\"type\":\"ConnectorPlacement.EquallySpacedRectSide\",\"uuid\":\"1cbb86fd-02d7-4865-80eb-cfab46dca279\"},{\"content\":{\"connectorIds\":[\"In1\"],\"side\":\"BOTTOM\"},\"type\":\"ConnectorPlacement.EquallySpacedRectSide\",\"uuid\":\"666c5156-ac3a-4b1c-905d-ea8e134facab\"}]},\"type\":\"ConnectorPlacement.EquallySpacedConnector\",\"uuid\":\"62703e30-84e5-4f8f-9fd6-529661229832\"}],\"packageUris\":[\"http://schema.mathworks.com/mf0/Connector/R2020b\"],\"version\":\"1.0\"}"
  jtoeFR : sm_lib/Joints/Weld Joint  JointMode=Normal  CompositeWrenchDir=FollowerOnBase  CompositeWrenchFrame=BaseFrame  SenseConstraintForce=off  SenseConstraintTorque=off  SenseTotalForce=off  SenseTotalTorque=off
  toeFR : Subsystem
  Conn1 : PMIOPort  Side=Left
  G : PMIOPort  Port=2  Side=Left
  meas : Outport  VectorParamsAs1DForOutWhenUnconnected=off
  wires:
  Bus Creator/1 -> meas/1
  toeFR/1(Fn) -> Bus Creator/4
  toeFR/2(Ff) -> Bus Creator/5
  Subsystem/1(Sensor) -> Bus Creator/1
  Subsystem1/1(Sensor) -> Bus Creator/2
  Subsystem2/1(Sensor) -> Bus Creator/3
  Gain2/1 -> Subsystem2/1(torque)
  InputFB/1 -> Demux/1
  Demux/1 -> Gain/1  "torque"
  Demux/2 -> Gain1/1  "torque"
  Demux/3 -> Gain2/1  "torque"
  Gain1/1 -> Subsystem1/1(torque)
  Gain/1 -> Subsystem/1(torque)
  connections:
  jtoeFR/RConn1 -- toeFR/LConn1
  FR_lower_leg/RConn1 -- jtoeFR/LConn1
  Subsystem/LConn1 -- Conn1/RConn1
  FR_hip_motor/LConn1 -- Subsystem/RConn1
  G/RConn1 -- toeFR/RConn1
  FR_upper_leg/LConn1 -- Subsystem1/RConn1
  FR_hip_motor/RConn1 -- Subsystem1/LConn1
  Subsystem2/LConn1 -- FR_upper_leg/RConn1
  FR_lower_leg/LConn1 -- Subsystem2/RConn1

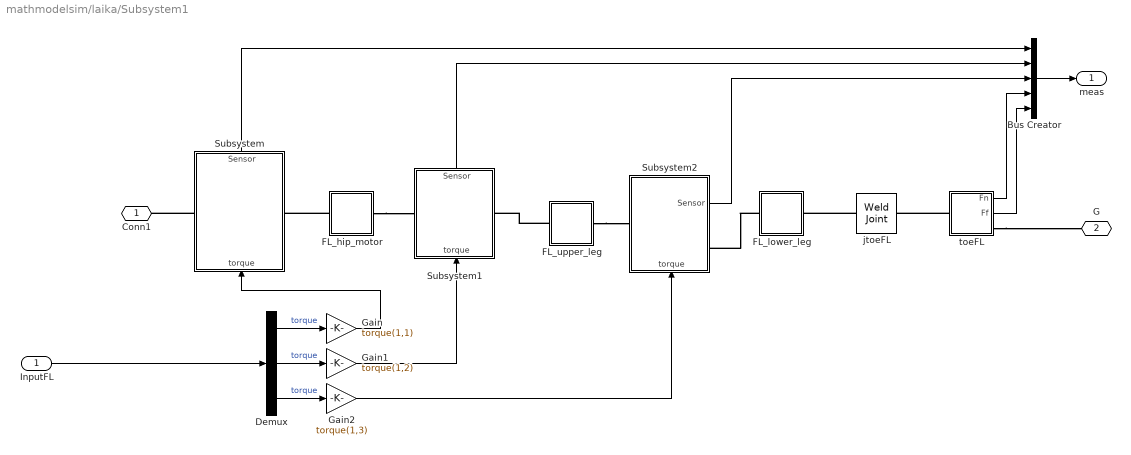
== system mathmodelsim/laika/Subsystem1 ==
  InputFL : Inport
  Bus Creator : BusCreator  Inputs=5
  Demux : Demux  Outputs=3
  FL_hip_motor : Subsystem
  FL_lower_leg : Subsystem
  FL_upper_leg : Subsystem
  Gain : Gain  Gain=torque(1,1)
  Gain1 : Gain  Gain=torque(1,2)
  Gain2 : Gain  Gain=torque(1,3)
  Subsystem : Subsystem
      settings: PortSchema="{\"entries\":[{\"content\":{\"sides\":[{\"content\":{\"connectorIds\":[\"LConn1\"]},\"type\":\"ConnectorPlacement.EquallySpacedRectSide\",\"uuid\":\"d10d1646-662a-418c-8f44-f8cb7d7b2586\"},{\"content\":{\"connectorIds\":[\"RConn1\"],\"side\":\"RIGHT\"},\"type\":\"ConnectorPlacement.EquallySpacedRectSide\",\"uuid\":\"1df4eb92-be91-4006-ac5e-dec2e273d2b2\"},{\"content\":{\"connectorIds\":[\"Out1\"],\"side\":\"TOP\"},\"type\":\"ConnectorPlacement.EquallySpacedRectSide\",\"uuid\":\"1cbb86fd-02d7-4865-80eb-cfab46dca279\"},{\"content\":{\"connectorIds\":[\"In1\"],\"side\":\"BOTTOM\"},\"type\":\"ConnectorPlacement.EquallySpacedRectSide\",\"uuid\":\"c11095bb-d672-4e30-a4ef-8f5c7235aabe\"}]},\"type\":\"ConnectorPlacement.EquallySpacedConnector\",\"uuid\":\"62703e30-84e5-4f8f-9fd6-529661229832\"}],\"packageUris\":[\"http://schema.mathworks.com/mf0/Connector/R2020b\"],\"version\":\"1.0\"}"
  Subsystem1 : Subsystem
      settings: PortSchema="{\"entries\":[{\"content\":{\"sides\":[{\"content\":{\"connectorIds\":[\"LConn1\"]},\"type\":\"ConnectorPlacement.EquallySpacedRectSide\",\"uuid\":\"d10d1646-662a-418c-8f44-f8cb7d7b2586\"},{\"content\":{\"connectorIds\":[\"RConn1\"],\"side\":\"RIGHT\"},\"type\":\"ConnectorPlacement.EquallySpacedRectSide\",\"uuid\":\"1df4eb92-be91-4006-ac5e-dec2e273d2b2\"},{\"content\":{\"connectorIds\":[\"Out1\"],\"side\":\"TOP\"},\"type\":\"ConnectorPlacement.EquallySpacedRectSide\",\"uuid\":\"1cbb86fd-02d7-4865-80eb-cfab46dca279\"},{\"content\":{\"connectorIds\":[\"In1\"],\"side\":\"BOTTOM\"},\"type\":\"ConnectorPlacement.EquallySpacedRectSide\",\"uuid\":\"8bee2df4-a927-4cf9-9983-bdcad833a156\"}]},\"type\":\"ConnectorPlacement.EquallySpacedConnector\",\"uuid\":\"62703e30-84e5-4f8f-9fd6-529661229832\"}],\"packageUris\":[\"http://schema.mathworks.com/mf0/Connector/R2020b\"],\"version\":\"1.0\"}"
  Subsystem2 : Subsystem
      settings: PortSchema="{\"entries\":[{\"content\":{\"sides\":[{\"content\":{\"connectorIds\":[\"LConn1\"]},\"type\":\"ConnectorPlacement.EquallySpacedRectSide\",\"uuid\":\"d10d1646-662a-418c-8f44-f8cb7d7b2586\"},{\"content\":{\"connectorIds\":[\"Out1\",\"RConn1\"],\"side\":\"RIGHT\"},\"type\":\"ConnectorPlacement.EquallySpacedRectSide\",\"uuid\":\"1df4eb92-be91-4006-ac5e-dec2e273d2b2\"},{\"content\":{\"side\":\"TOP\"},\"type\":\"ConnectorPlacement.EquallySpacedRectSide\",\"uuid\":\"1cbb86fd-02d7-4865-80eb-cfab46dca279\"},{\"content\":{\"connectorIds\":[\"In1\"],\"side\":\"BOTTOM\"},\"type\":\"ConnectorPlacement.EquallySpacedRectSide\",\"uuid\":\"666c5156-ac3a-4b1c-905d-ea8e134facab\"}]},\"type\":\"ConnectorPlacement.EquallySpacedConnector\",\"uuid\":\"62703e30-84e5-4f8f-9fd6-529661229832\"}],\"packageUris\":[\"http://schema.mathworks.com/mf0/Connector/R2020b\"],\"version\":\"1.0\"}"
  jtoeFL : sm_lib/Joints/Weld Joint  JointMode=Normal  CompositeWrenchDir=FollowerOnBase  CompositeWrenchFrame=BaseFrame  SenseConstraintForce=off  SenseConstraintTorque=off  SenseTotalForce=off  SenseTotalTorque=off
  toeFL : Subsystem
  Conn1 : PMIOPort  Side=Left
  G : PMIOPort  Port=2  Side=Left
  meas : Outport  VectorParamsAs1DForOutWhenUnconnected=off
  wires:
  Subsystem1/1(Sensor) -> Bus Creator/2
  Subsystem/1(Sensor) -> Bus Creator/1
  toeFL/1(Fn) -> Bus Creator/4
  toeFL/2(Ff) -> Bus Creator/5
  Bus Creator/1 -> meas/1
  Subsystem2/1(Sensor) -> Bus Creator/3
  Gain2/1 -> Subsystem2/1(torque)
  InputFL/1 -> Demux/1
  Demux/1 -> Gain/1  "torque"
  Demux/2 -> Gain1/1  "torque"
  Demux/3 -> Gain2/1  "torque"
  Gain1/1 -> Subsystem1/1(torque)
  Gain/1 -> Subsystem/1(torque)
  connections:
  toeFL/LConn1 -- jtoeFL/RConn1
  jtoeFL/LConn1 -- FL_lower_leg/RConn1
  FL_upper_leg/LConn1 -- Subsystem1/RConn1
  FL_hip_motor/LConn1 -- Subsystem/RConn1
  FL_lower_leg/LConn1 -- Subsystem2/RConn1
  Subsystem/LConn1 -- Conn1/RConn1
  FL_upper_leg/RConn1 -- Subsystem2/LConn1
  FL_hip_motor/RConn1 -- Subsystem1/LConn1
  toeFL/RConn1 -- G/RConn1
